simulink model "d5_a_2_model"  (R2025a)
settings: Solver=VariableStepAuto  StartTime=0.0  StopTime=10.0  RelTol=1e-3
values from neighbouring files (symbols this model uses):
  A = Gp.Denominator{1,1}    [d5_RST.m]    (also in d5_a_1.m = Gpk.Denominator{1,1}; d5_a_2.m = Gpk.Denominator{1,1}; d5_b_1.m = Gpd.Denominator{1,1})
  B = Gp.Numerator{1,1}    [d5_RST.m]    (also in d5_a_1.m = Gpk.Numerator{1,1}; d5_a_2.m = Gpk.Numerator{1,1}; d5_b_1.m = Gpd.Numerator{1,1})
  Rk = [1, RS(1), 0]    [d5_a_1.m]    (also in d5_a_2.m = [1, RS(1), w^2, w^2 * RS(1)])
  Sk = RS(2:end)'    [d5_a_1.m]    (also in d5_a_2.m)
  Tsk = 1 / dcgain(1/Rsk * feedback(Gpk, Ssk/Rsk))    [d5_a_1.m]    (also in d5_a_2.m)
  w = 1    [d5_a_2.m]    (also in d5_b_2.m)
settings Model: Creator=Korisnik  LastModifiedBy=Korisnik

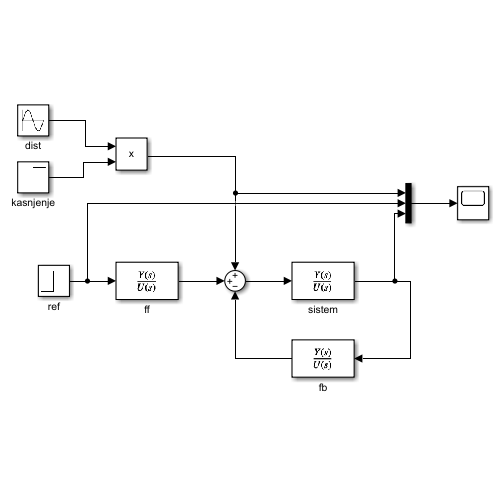
[thumbnail: Simulink's stored preview of the top-level diagram]
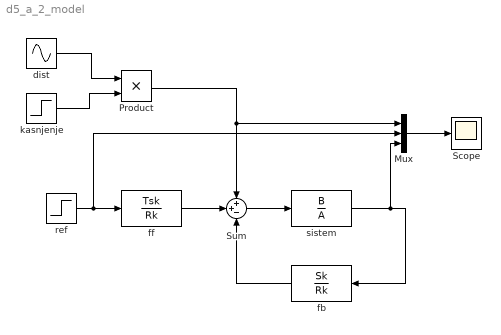
== system d5_a_2_model ==
  Mux : Mux  Inputs=3
  Product : Product
  Scope : Scope
      settings: ActiveDisplayYMinimum=-12.476137212091782  ActiveDisplayYMaximum=12.4926388074398
  Sum : Sum  Inputs=++-
  dist : Sin  Amplitude=10  Frequency=w  SampleTime=0
  fb : TransferFcn  Numerator=Sk  Denominator=Rk
  ff : TransferFcn  Numerator=Tsk  Denominator=Rk
  kasnjenje : Step  Time=3  SampleTime=0
  ref : Step  Time=0  After=8  SampleTime=0
  sistem : TransferFcn  Numerator=B  Denominator=A
  wires:
  sistem/1 -> Mux/3, fb/1
  ff/1 -> Sum/2
  ref/1 -> Mux/2, ff/1
  fb/1 -> Sum/3
  Sum/1 -> sistem/1
  Mux/1 -> Scope/1
  dist/1 -> Product/1
  kasnjenje/1 -> Product/2
  Product/1 -> Mux/1, Sum/1
